simulink subsystem "Baroreflex_TPR"  (R2023b)
settings: Solver=VariableStepAuto  StartTime=0.0  StopTime=10.0  RelTol=1e-3
values from neighbouring files (symbols this model uses):
  b = 0.01    [Project2024_params_Group3.m]
  T_D = 0.002    [Project2024_params_Group3.m]
  tau_2 = 0.01    [Project2024_params_Group3.m]
  TPR_eq = 12.5    [Project2024_params_Group3.m]    (also in compute_indices.m = mean(TPR_data(pre_infusion_indices)))
settings Model: Creator=jamesyeh  LastModifiedBy=jamesyeh

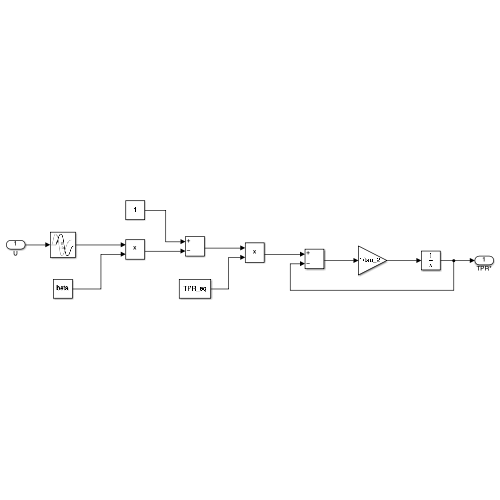
[thumbnail: Simulink's stored preview of the top-level diagram]
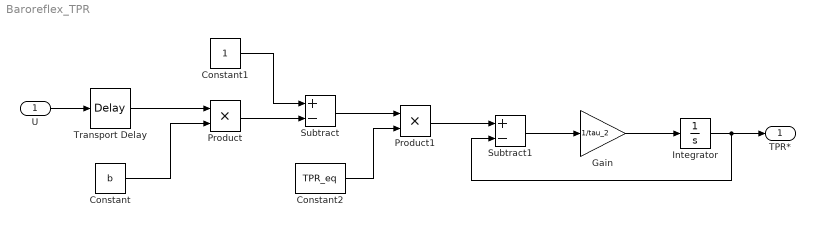
== system Baroreflex_TPR ==
  U : Inport
  Constant : Constant  Value=b
  Constant1 : Constant
  Constant2 : Constant  Value=TPR_eq
  Gain : Gain  Gain=1/tau_2
  Integrator : Integrator
  Product : Product
  Product1 : Product
  Subtract : Sum  Inputs=+-
  Subtract1 : Sum  Inputs=+-
  Transport Delay : TransportDelay  DelayTime=T_D
  TPR* : Outport
  wires:
  U/1 -> Transport Delay/1
  Transport Delay/1 -> Product/1
  Constant/1 -> Product/2
  Constant1/1 -> Subtract/1
  Product/1 -> Subtract/2
  Subtract/1 -> Product1/1
  Constant2/1 -> Product1/2
  Product1/1 -> Subtract1/1
  Subtract1/1 -> Gain/1
  Gain/1 -> Integrator/1
  Integrator/1 -> Subtract1/2, TPR*/1
